simulink library "VISMODAL_MASTER"  (Simulink 8.6)
settings: Solver=VariableStepAuto  StartTime=0.0  StopTime=10.0  RelTol=1e-3
libraries: VIS_LIB x140, cdsFilt x34, cdsMuxMatrix x6, VISMODAL_MASTER x1
(part 3 of 5)

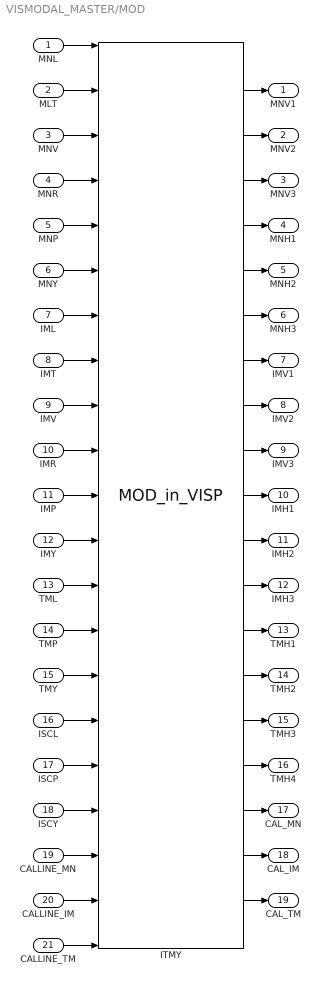
== system VISMODAL_MASTER/MOD ==
  MNL : Inport
  MLT : Inport  Port=2
  MNV : Inport  Port=3
  MNR : Inport  Port=4
  MNP : Inport  Port=5
  MNY : Inport  Port=6
  IML : Inport  Port=7
  IMT : Inport  Port=8
  IMV : Inport  Port=9
  IMR : Inport  Port=10
  IMP : Inport  Port=11
  IMY : Inport  Port=12
  TML : Inport  Port=13
  TMP : Inport  Port=14
  TMY : Inport  Port=15
  ISCL : Inport  Port=16
  ISCP : Inport  Port=17
  ISCY : Inport  Port=18
  CALLINE_MN : Inport  Port=19
  CALLINE_IM : Inport  Port=20
  CALLINE_TM : Inport  Port=21
  ITMY : VIS_LIB/MODAL/MOD_in_VISP  Tag=top_names
  MNV1 : Outport
  MNV2 : Outport  Port=2
  MNV3 : Outport  Port=3
  MNH1 : Outport  Port=4
  MNH2 : Outport  Port=5
  MNH3 : Outport  Port=6
  IMV1 : Outport  Port=7
  IMV2 : Outport  Port=8
  IMV3 : Outport  Port=9
  IMH1 : Outport  Port=10
  IMH2 : Outport  Port=11
  IMH3 : Outport  Port=12
  TMH1 : Outport  Port=13
  TMH2 : Outport  Port=14
  TMH3 : Outport  Port=15
  TMH4 : Outport  Port=16
  CAL_MN : Outport  Port=17
  CAL_IM : Outport  Port=18
  CAL_TM : Outport  Port=19
  wires:
  MNL/1 -> ITMY/1
  TMY/1 -> ITMY/15
  MLT/1 -> ITMY/2
  MNV/1 -> ITMY/3
  MNR/1 -> ITMY/4
  MNP/1 -> ITMY/5
  MNY/1 -> ITMY/6
  IML/1 -> ITMY/7
  IMT/1 -> ITMY/8
  IMV/1 -> ITMY/9
  IMR/1 -> ITMY/10
  IMP/1 -> ITMY/11
  IMY/1 -> ITMY/12
  TML/1 -> ITMY/13
  TMP/1 -> ITMY/14
  ITMY/1 -> MNV1/1
  ITMY/16 -> TMH4/1
  ITMY/2 -> MNV2/1
  ITMY/3 -> MNV3/1
  ITMY/4 -> MNH1/1
  ITMY/5 -> MNH2/1
  ITMY/6 -> MNH3/1
  ITMY/7 -> IMV1/1
  ITMY/8 -> IMV2/1
  ITMY/9 -> IMV3/1
  ITMY/10 -> IMH1/1
  ITMY/11 -> IMH2/1
  ITMY/12 -> IMH3/1
  ITMY/13 -> TMH1/1
  ITMY/14 -> TMH2/1
  ITMY/15 -> TMH3/1
  ISCL/1 -> ITMY/16
  CALLINE_TM/1 -> ITMY/21
  CALLINE_IM/1 -> ITMY/20
  CALLINE_MN/1 -> ITMY/19
  ISCP/1 -> ITMY/17
  ISCY/1 -> ITMY/18
  ITMY/17 -> CAL_MN/1
  ITMY/18 -> CAL_IM/1
  ITMY/19 -> CAL_TM/1

== system VISMODAL_MASTER/ITMY/AI_GAS ==
  note: #DAQ Channels
      |
      | M1_OUT 256
      | M2_OUT 256
      | M3_OUT 256
      | M4_OUT 256
      | M5_OUT 256
  M1_IN : Inport
  M2_IN : Inport  Port=2
  M3_IN : Inport  Port=3
  M4_IN : Inport  Port=4
  M5_IN : Inport  Port=5
  M1 : cdsFilt/Subsystem  Tag=cdsFilt  Description=|
      | Purpose:                                                                                                                                                                                                                                  
      | Standard CDS IIR filter module.                                                                                                                                                                                                           
      |                                                                                                                                                                                                                                           
      | Operation:                                                                                                                                                                                                                                
      | Consists of 10 second order section IIR filters, plus a ramped gain stage. In FE code, also provides pre-defined test points and excitation channel inputs. The filter coefficients are defined in the LIGO system using the 'foton' tool.
      |                                                                                                                                                                                                                                           
      | Usage:                                                                                                                                                                                                                                    
      | Name the part with the desired filter module name.
      settings: AttributesFormatString=%<Tag>
  M2 : cdsFilt/Subsystem  Tag=cdsFilt  Description=|
      | Purpose:                                                                                                                                                                                                                                  
      | Standard CDS IIR filter module.                                                                                                                                                                                                           
      |                                                                                                                                                                                                                                           
      | Operation:                                                                                                                                                                                                                                
      | Consists of 10 second order section IIR filters, plus a ramped gain stage. In FE code, also provides pre-defined test points and excitation channel inputs. The filter coefficients are defined in the LIGO system using the 'foton' tool.
      |                                                                                                                                                                                                                                           
      | Usage:                                                                                                                                                                                                                                    
      | Name the part with the desired filter module name.
      settings: AttributesFormatString=%<Tag>
  M3 : cdsFilt/Subsystem  Tag=cdsFilt  Description=|
      | Purpose:                                                                                                                                                                                                                                  
      | Standard CDS IIR filter module.                                                                                                                                                                                                           
      |                                                                                                                                                                                                                                           
      | Operation:                                                                                                                                                                                                                                
      | Consists of 10 second order section IIR filters, plus a ramped gain stage. In FE code, also provides pre-defined test points and excitation channel inputs. The filter coefficients are defined in the LIGO system using the 'foton' tool.
      |                                                                                                                                                                                                                                           
      | Usage:                                                                                                                                                                                                                                    
      | Name the part with the desired filter module name.
      settings: AttributesFormatString=%<Tag>
  M4 : cdsFilt/Subsystem  Tag=cdsFilt  Description=|
      | Purpose:                                                                                                                                                                                                                                  
      | Standard CDS IIR filter module.                                                                                                                                                                                                           
      |                                                                                                                                                                                                                                           
      | Operation:                                                                                                                                                                                                                                
      | Consists of 10 second order section IIR filters, plus a ramped gain stage. In FE code, also provides pre-defined test points and excitation channel inputs. The filter coefficients are defined in the LIGO system using the 'foton' tool.
      |                                                                                                                                                                                                                                           
      | Usage:                                                                                                                                                                                                                                    
      | Name the part with the desired filter module name.
      settings: AttributesFormatString=%<Tag>
  M5 : cdsFilt/Subsystem  Tag=cdsFilt  Description=|
      | Purpose:                                                                                                                                                                                                                                  
      | Standard CDS IIR filter module.                                                                                                                                                                                                           
      |                                                                                                                                                                                                                                           
      | Operation:                                                                                                                                                                                                                                
      | Consists of 10 second order section IIR filters, plus a ramped gain stage. In FE code, also provides pre-defined test points and excitation channel inputs. The filter coefficients are defined in the LIGO system using the 'foton' tool.
      |                                                                                                                                                                                                                                           
      | Usage:                                                                                                                                                                                                                                    
      | Name the part with the desired filter module name.
      settings: AttributesFormatString=%<Tag>
  M1_OUT : Outport
  M2_OUT : Outport  Port=2
  M3_OUT : Outport  Port=3
  M4_OUT : Outport  Port=4
  M5_OUT : Outport  Port=5
  wires:
  M3/1 -> M3_OUT/1
  M2/1 -> M2_OUT/1
  M4/1 -> M4_OUT/1
  M5/1 -> M5_OUT/1
  M1/1 -> M1_OUT/1
  M1_IN/1 -> M1/1
  M2_IN/1 -> M2/1
  M3_IN/1 -> M3/1
  M4_IN/1 -> M4/1
  M5_IN/1 -> M5/1

== system VISMODAL_MASTER/ITMY/COILOUT_GAS ==
  note: #DAQ Channels
      |
      | F0_OUT 256
      | F1_OUT 256
      | F2_OUT 256
      | F3_OUT 256
      | BF_OUT 256
  F0_IN : Inport
  F1_IN : Inport  Port=2
  F2_IN : Inport  Port=3
  F3_IN : Inport  Port=4
  BF_IN : Inport  Port=5
  BF : cdsFilt/Subsystem  Tag=cdsFilt  Description=|
      | Purpose:                                                                                                                                                                                                                                  
      | Standard CDS IIR filter module.                                                                                                                                                                                                           
      |                                                                                                                                                                                                                                           
      | Operation:                                                                                                                                                                                                                                
      | Consists of 10 second order section IIR filters, plus a ramped gain stage. In FE code, also provides pre-defined test points and excitation channel inputs. The filter coefficients are defined in the LIGO system using the 'foton' tool.
      |                                                                                                                                                                                                                                           
      | Usage:                                                                                                                                                                                                                                    
      | Name the part with the desired filter module name.
      settings: AttributesFormatString=%<Tag>
  F0 : cdsFilt/Subsystem  Tag=cdsFilt  Description=|
      | Purpose:                                                                                                                                                                                                                                  
      | Standard CDS IIR filter module.                                                                                                                                                                                                           
      |                                                                                                                                                                                                                                           
      | Operation:                                                                                                                                                                                                                                
      | Consists of 10 second order section IIR filters, plus a ramped gain stage. In FE code, also provides pre-defined test points and excitation channel inputs. The filter coefficients are defined in the LIGO system using the 'foton' tool.
      |                                                                                                                                                                                                                                           
      | Usage:                                                                                                                                                                                                                                    
      | Name the part with the desired filter module name.
      settings: AttributesFormatString=%<Tag>
  F1 : cdsFilt/Subsystem  Tag=cdsFilt  Description=|
      | Purpose:                                                                                                                                                                                                                                  
      | Standard CDS IIR filter module.                                                                                                                                                                                                           
      |                                                                                                                                                                                                                                           
      | Operation:                                                                                                                                                                                                                                
      | Consists of 10 second order section IIR filters, plus a ramped gain stage. In FE code, also provides pre-defined test points and excitation channel inputs. The filter coefficients are defined in the LIGO system using the 'foton' tool.
      |                                                                                                                                                                                                                                           
      | Usage:                                                                                                                                                                                                                                    
      | Name the part with the desired filter module name.
      settings: AttributesFormatString=%<Tag>
  F2 : cdsFilt/Subsystem  Tag=cdsFilt  Description=|
      | Purpose:                                                                                                                                                                                                                                  
      | Standard CDS IIR filter module.                                                                                                                                                                                                           
      |                                                                                                                                                                                                                                           
      | Operation:                                                                                                                                                                                                                                
      | Consists of 10 second order section IIR filters, plus a ramped gain stage. In FE code, also provides pre-defined test points and excitation channel inputs. The filter coefficients are defined in the LIGO system using the 'foton' tool.
      |                                                                                                                                                                                                                                           
      | Usage:                                                                                                                                                                                                                                    
      | Name the part with the desired filter module name.
      settings: AttributesFormatString=%<Tag>
  F3 : cdsFilt/Subsystem  Tag=cdsFilt  Description=|
      | Purpose:                                                                                                                                                                                                                                  
      | Standard CDS IIR filter module.                                                                                                                                                                                                           
      |                                                                                                                                                                                                                                           
      | Operation:                                                                                                                                                                                                                                
      | Consists of 10 second order section IIR filters, plus a ramped gain stage. In FE code, also provides pre-defined test points and excitation channel inputs. The filter coefficients are defined in the LIGO system using the 'foton' tool.
      |                                                                                                                                                                                                                                           
      | Usage:                                                                                                                                                                                                                                    
      | Name the part with the desired filter module name.
      settings: AttributesFormatString=%<Tag>
  F0_OUT : Outport
  F1_OUT : Outport  Port=2
  F2_OUT : Outport  Port=3
  F3_OUT : Outport  Port=4
  BF_OUT : Outport  Port=5
  wires:
  F2/1 -> F2_OUT/1
  F1/1 -> F1_OUT/1
  F3/1 -> F3_OUT/1
  BF/1 -> BF_OUT/1
  F0/1 -> F0_OUT/1
  F0_IN/1 -> F0/1
  F1_IN/1 -> F1/1
  F2_IN/1 -> F2/1
  F3_IN/1 -> F3/1
  BF_IN/1 -> BF/1

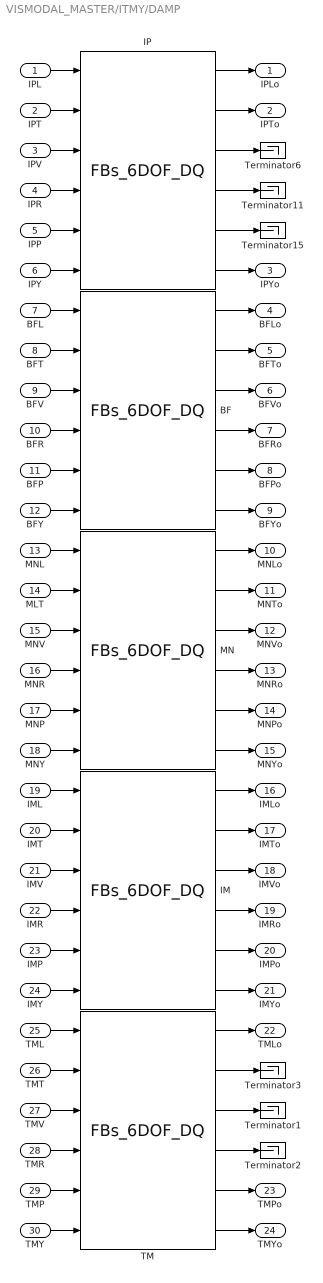
== system VISMODAL_MASTER/ITMY/DAMP ==
  IPL : Inport
  IPT : Inport  Port=2
  IPV : Inport  Port=3
  IPR : Inport  Port=4
  IPP : Inport  Port=5
  IPY : Inport  Port=6
  BFL : Inport  Port=7
  BFT : Inport  Port=8
  BFV : Inport  Port=9
  BFR : Inport  Port=10
  BFP : Inport  Port=11
  BFY : Inport  Port=12
  MNL : Inport  Port=13
  MLT : Inport  Port=14
  MNV : Inport  Port=15
  MNR : Inport  Port=16
  MNP : Inport  Port=17
  MNY : Inport  Port=18
  IML : Inport  Port=19
  IMT : Inport  Port=20
  IMV : Inport  Port=21
  IMR : Inport  Port=22
  IMP : Inport  Port=23
  IMY : Inport  Port=24
  TML : Inport  Port=25
  TMT : Inport  Port=26
  TMV : Inport  Port=27
  TMR : Inport  Port=28
  TMP : Inport  Port=29
  TMY : Inport  Port=30
  BF : VIS_LIB/UTILs/FBs_6DOF_DQ
  IM : VIS_LIB/UTILs/FBs_6DOF_DQ
  IP : VIS_LIB/UTILs/FBs_6DOF_DQ
  MN : VIS_LIB/UTILs/FBs_6DOF_DQ
  TM : VIS_LIB/UTILs/FBs_6DOF_DQ
  Terminator{1..3,6,11,15} (6 alike) : Terminator
  IPLo : Outport
  IPTo : Outport  Port=2
  IPYo : Outport  Port=3
  BFLo : Outport  Port=4
  BFTo : Outport  Port=5
  BFVo : Outport  Port=6
  BFRo : Outport  Port=7
  BFPo : Outport  Port=8
  BFYo : Outport  Port=9
  MNLo : Outport  Port=10
  MNTo : Outport  Port=11
  MNVo : Outport  Port=12
  MNRo : Outport  Port=13
  MNPo : Outport  Port=14
  MNYo : Outport  Port=15
  IMLo : Outport  Port=16
  IMTo : Outport  Port=17
  IMVo : Outport  Port=18
  IMRo : Outport  Port=19
  IMPo : Outport  Port=20
  IMYo : Outport  Port=21
  TMLo : Outport  Port=22
  TMPo : Outport  Port=23
  TMYo : Outport  Port=24
  wires:
  IPL/1 -> IP/1
  IPT/1 -> IP/2
  IPY/1 -> IP/6
  BFL/1 -> BF/1
  BFT/1 -> BF/2
  BFV/1 -> BF/3
  BFR/1 -> BF/4
  BFP/1 -> BF/5
  BFY/1 -> BF/6
  IPV/1 -> IP/3
  IPR/1 -> IP/4
  IPP/1 -> IP/5
  MNL/1 -> MN/1
  TMY/1 -> TM/6
  MLT/1 -> MN/2
  MNV/1 -> MN/3
  MNR/1 -> MN/4
  MNP/1 -> MN/5
  MNY/1 -> MN/6
  IML/1 -> IM/1
  IMT/1 -> IM/2
  IMV/1 -> IM/3
  IMR/1 -> IM/4
  IMP/1 -> IM/5
  IMY/1 -> IM/6
  TML/1 -> TM/1
  TMP/1 -> TM/5
  TMV/1 -> TM/3
  TMT/1 -> TM/2
  TMR/1 -> TM/4
  IP/1 -> IPLo/1
  IP/2 -> IPTo/1
  IP/6 -> IPYo/1
  BF/1 -> BFLo/1
  BF/2 -> BFTo/1
  BF/3 -> BFVo/1
  BF/4 -> BFRo/1
  BF/5 -> BFPo/1
  BF/6 -> BFYo/1
  MN/1 -> MNLo/1
  MN/2 -> MNTo/1
  MN/3 -> MNVo/1
  MN/4 -> MNRo/1
  MN/5 -> MNPo/1
  MN/6 -> MNYo/1
  IM/1 -> IMLo/1
  IM/2 -> IMTo/1
  IM/3 -> IMVo/1
  IM/4 -> IMRo/1
  IM/5 -> IMPo/1
  IM/6 -> IMYo/1
  TM/5 -> TMPo/1
  TM/6 -> TMYo/1
  TM/1 -> TMLo/1
  IP/3 -> Terminator6/1
  IP/5 -> Terminator15/1
  IP/4 -> Terminator11/1
  TM/2 -> Terminator3/1
  TM/4 -> Terminator2/1
  TM/3 -> Terminator1/1

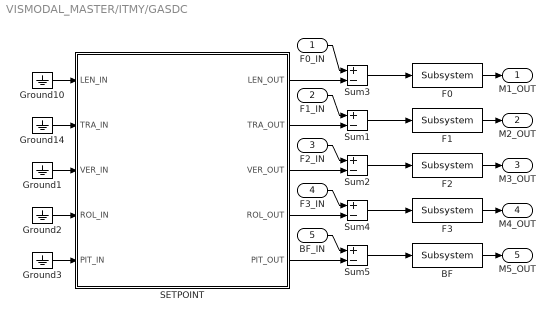
== system VISMODAL_MASTER/ITMY/GASDC ==
  F0_IN : Inport
  F1_IN : Inport  Port=2
  F2_IN : Inport  Port=3
  F3_IN : Inport  Port=4
  BF_IN : Inport  Port=5
  BF : cdsFilt/Subsystem  Tag=cdsFilt  Description=|
      | Purpose:                                                                                                                                                                                                                                  
      | Standard CDS IIR filter module.                                                                                                                                                                                                           
      |                                                                                                                                                                                                                                           
      | Operation:                                                                                                                                                                                                                                
      | Consists of 10 second order section IIR filters, plus a ramped gain stage. In FE code, also provides pre-defined test points and excitation channel inputs. The filter coefficients are defined in the LIGO system using the 'foton' tool.
      |                                                                                                                                                                                                                                           
      | Usage:                                                                                                                                                                                                                                    
      | Name the part with the desired filter module name.
      settings: AttributesFormatString=%<Tag>
  F0 : cdsFilt/Subsystem  Tag=cdsFilt  Description=|
      | Purpose:                                                                                                                                                                                                                                  
      | Standard CDS IIR filter module.                                                                                                                                                                                                           
      |                                                                                                                                                                                                                                           
      | Operation:                                                                                                                                                                                                                                
      | Consists of 10 second order section IIR filters, plus a ramped gain stage. In FE code, also provides pre-defined test points and excitation channel inputs. The filter coefficients are defined in the LIGO system using the 'foton' tool.
      |                                                                                                                                                                                                                                           
      | Usage:                                                                                                                                                                                                                                    
      | Name the part with the desired filter module name.
      settings: AttributesFormatString=%<Tag>
  F1 : cdsFilt/Subsystem  Tag=cdsFilt  Description=|
      | Purpose:                                                                                                                                                                                                                                  
      | Standard CDS IIR filter module.                                                                                                                                                                                                           
      |                                                                                                                                                                                                                                           
      | Operation:                                                                                                                                                                                                                                
      | Consists of 10 second order section IIR filters, plus a ramped gain stage. In FE code, also provides pre-defined test points and excitation channel inputs. The filter coefficients are defined in the LIGO system using the 'foton' tool.
      |                                                                                                                                                                                                                                           
      | Usage:                                                                                                                                                                                                                                    
      | Name the part with the desired filter module name.
      settings: AttributesFormatString=%<Tag>
  F2 : cdsFilt/Subsystem  Tag=cdsFilt  Description=|
      | Purpose:                                                                                                                                                                                                                                  
      | Standard CDS IIR filter module.                                                                                                                                                                                                           
      |                                                                                                                                                                                                                                           
      | Operation:                                                                                                                                                                                                                                
      | Consists of 10 second order section IIR filters, plus a ramped gain stage. In FE code, also provides pre-defined test points and excitation channel inputs. The filter coefficients are defined in the LIGO system using the 'foton' tool.
      |                                                                                                                                                                                                                                           
      | Usage:                                                                                                                                                                                                                                    
      | Name the part with the desired filter module name.
      settings: AttributesFormatString=%<Tag>
  F3 : cdsFilt/Subsystem  Tag=cdsFilt  Description=|
      | Purpose:                                                                                                                                                                                                                                  
      | Standard CDS IIR filter module.                                                                                                                                                                                                           
      |                                                                                                                                                                                                                                           
      | Operation:                                                                                                                                                                                                                                
      | Consists of 10 second order section IIR filters, plus a ramped gain stage. In FE code, also provides pre-defined test points and excitation channel inputs. The filter coefficients are defined in the LIGO system using the 'foton' tool.
      |                                                                                                                                                                                                                                           
      | Usage:                                                                                                                                                                                                                                    
      | Name the part with the desired filter module name.
      settings: AttributesFormatString=%<Tag>
  Ground{1..3,10,14} (5 alike) : Ground
  SETPOINT : Subsystem
  Sum{1..5} (5 alike) : Sum  Inputs=+-
  M1_OUT : Outport
  M2_OUT : Outport  Port=2
  M3_OUT : Outport  Port=3
  M4_OUT : Outport  Port=4
  M5_OUT : Outport  Port=5
  wires:
  F2/1 -> M3_OUT/1
  F1/1 -> M2_OUT/1
  F3/1 -> M4_OUT/1
  BF/1 -> M5_OUT/1
  F0/1 -> M1_OUT/1
  Ground10/1 -> SETPOINT/1(LEN_IN)
  Ground14/1 -> SETPOINT/2(TRA_IN)
  Ground1/1 -> SETPOINT/3(VER_IN)
  Ground2/1 -> SETPOINT/4(ROL_IN)
  Ground3/1 -> SETPOINT/5(PIT_IN)
  F0_IN/1 -> Sum3/1
  SETPOINT/1(LEN_OUT) -> Sum3/2
  Sum3/1 -> F0/1
  SETPOINT/2(TRA_OUT) -> Sum1/2
  Sum1/1 -> F1/1
  F1_IN/1 -> Sum1/1
  SETPOINT/3(VER_OUT) -> Sum2/2
  F2_IN/1 -> Sum2/1
  Sum2/1 -> F2/1
  SETPOINT/4(ROL_OUT) -> Sum4/2
  F3_IN/1 -> Sum4/1
  Sum4/1 -> F3/1
  Sum5/1 -> BF/1
  BF_IN/1 -> Sum5/1
  SETPOINT/5(PIT_OUT) -> Sum5/2

== system VISMODAL_MASTER/ITMY/IPDC ==
  IPL : Inport
  IPT : Inport  Port=2
  IPY : Inport  Port=3
  Ground1 : Ground
  Ground2 : Ground
  Ground3 : Ground
  LEN : cdsFilt/Subsystem  Tag=cdsFilt  Description=|
      | Purpose:                                                                                                                                                                                                                                  
      | Standard CDS IIR filter module.                                                                                                                                                                                                           
      |                                                                                                                                                                                                                                           
      | Operation:                                                                                                                                                                                                                                
      | Consists of 10 second order section IIR filters, plus a ramped gain stage. In FE code, also provides pre-defined test points and excitation channel inputs. The filter coefficients are defined in the LIGO system using the 'foton' tool.
      |                                                                                                                                                                                                                                           
      | Usage:                                                                                                                                                                                                                                    
      | Name the part with the desired filter module name.
      settings: AttributesFormatString=%<Tag>
  SETPOINT : Subsystem
  Sum1 : Sum  Inputs=+-
  Sum2 : Sum  Inputs=+-
  Sum3 : Sum  Inputs=+-
  TRA : cdsFilt/Subsystem  Tag=cdsFilt  Description=|
      | Purpose:                                                                                                                                                                                                                                  
      | Standard CDS IIR filter module.                                                                                                                                                                                                           
      |                                                                                                                                                                                                                                           
      | Operation:                                                                                                                                                                                                                                
      | Consists of 10 second order section IIR filters, plus a ramped gain stage. In FE code, also provides pre-defined test points and excitation channel inputs. The filter coefficients are defined in the LIGO system using the 'foton' tool.
      |                                                                                                                                                                                                                                           
      | Usage:                                                                                                                                                                                                                                    
      | Name the part with the desired filter module name.
      settings: AttributesFormatString=%<Tag>
  YAW : cdsFilt/Subsystem  Tag=cdsFilt  Description=|
      | Purpose:                                                                                                                                                                                                                                  
      | Standard CDS IIR filter module.                                                                                                                                                                                                           
      |                                                                                                                                                                                                                                           
      | Operation:                                                                                                                                                                                                                                
      | Consists of 10 second order section IIR filters, plus a ramped gain stage. In FE code, also provides pre-defined test points and excitation channel inputs. The filter coefficients are defined in the LIGO system using the 'foton' tool.
      |                                                                                                                                                                                                                                           
      | Usage:                                                                                                                                                                                                                                    
      | Name the part with the desired filter module name.
      settings: AttributesFormatString=%<Tag>
  LEN_OUT : Outport
  PIT_OUT : Outport  Port=2
  YAW_OUT : Outport  Port=3
  wires:
  IPL/1 -> Sum1/1
  SETPOINT/1(LEN_OUT) -> Sum1/2
  IPT/1 -> Sum2/1
  SETPOINT/2(PIT_OUT) -> Sum2/2
  Ground1/1 -> SETPOINT/1(LEN_IN)
  Ground3/1 -> SETPOINT/2(PIT_IN)
  TRA/1 -> PIT_OUT/1
  Sum2/1 -> TRA/1
  YAW/1 -> YAW_OUT/1
  Sum1/1 -> LEN/1
  LEN/1 -> LEN_OUT/1
  Ground2/1 -> SETPOINT/3(YAW_IN)
  IPY/1 -> Sum3/1
  Sum3/1 -> YAW/1
  SETPOINT/3(YAW_OUT) -> Sum3/2

== system VISMODAL_MASTER/ITMY/MNOL_SERVO_MN ==
  note: #DAQ Channels
      |
      | LEN_OUT 256
      | PIT_OUT 256
      | YAW_OUT 256
  LEN_IN : Inport
  PIT_IN : Inport  Port=2
  YAW_IN : Inport  Port=3
  LEN : cdsFilt/Subsystem  Tag=cdsFilt  Description=|
      | Purpose:                                                                                                                                                                                                                                  
      | Standard CDS IIR filter module.                                                                                                                                                                                                           
      |                                                                                                                                                                                                                                           
      | Operation:                                                                                                                                                                                                                                
      | Consists of 10 second order section IIR filters, plus a ramped gain stage. In FE code, also provides pre-defined test points and excitation channel inputs. The filter coefficients are defined in the LIGO system using the 'foton' tool.
      |                                                                                                                                                                                                                                           
      | Usage:                                                                                                                                                                                                                                    
      | Name the part with the desired filter module name.
      settings: AttributesFormatString=%<Tag>
  PIT : cdsFilt/Subsystem  Tag=cdsFilt  Description=|
      | Purpose:                                                                                                                                                                                                                                  
      | Standard CDS IIR filter module.                                                                                                                                                                                                           
      |                                                                                                                                                                                                                                           
      | Operation:                                                                                                                                                                                                                                
      | Consists of 10 second order section IIR filters, plus a ramped gain stage. In FE code, also provides pre-defined test points and excitation channel inputs. The filter coefficients are defined in the LIGO system using the 'foton' tool.
      |                                                                                                                                                                                                                                           
      | Usage:                                                                                                                                                                                                                                    
      | Name the part with the desired filter module name.
      settings: AttributesFormatString=%<Tag>
  YAW : cdsFilt/Subsystem  Tag=cdsFilt  Description=|
      | Purpose:                                                                                                                                                                                                                                  
      | Standard CDS IIR filter module.                                                                                                                                                                                                           
      |                                                                                                                                                                                                                                           
      | Operation:                                                                                                                                                                                                                                
      | Consists of 10 second order section IIR filters, plus a ramped gain stage. In FE code, also provides pre-defined test points and excitation channel inputs. The filter coefficients are defined in the LIGO system using the 'foton' tool.
      |                                                                                                                                                                                                                                           
      | Usage:                                                                                                                                                                                                                                    
      | Name the part with the desired filter module name.
      settings: AttributesFormatString=%<Tag>
  LEN_OUT : Outport
  PIT_OUT : Outport  Port=2
  YAW_OUT : Outport  Port=3
  wires:
  PIT/1 -> PIT_OUT/1
  PIT_IN/1 -> PIT/1
  YAW_IN/1 -> YAW/1
  YAW/1 -> YAW_OUT/1
  LEN_IN/1 -> LEN/1
  LEN/1 -> LEN_OUT/1
